simulink model "dsa2k_iwave_rfi"  (R2021a)
settings: Solver=VariableStepAuto  StartTime=0.0  StopTime=10.0  RelTol=1e-3
undefined symbols (not defined in the file): datetime, i, posixtime
libraries: xbsIndex_r4 x3053, casper_library_misc x61, rtr_casper_dsp_lib x31, xps_library x1
(part 4 of 43)

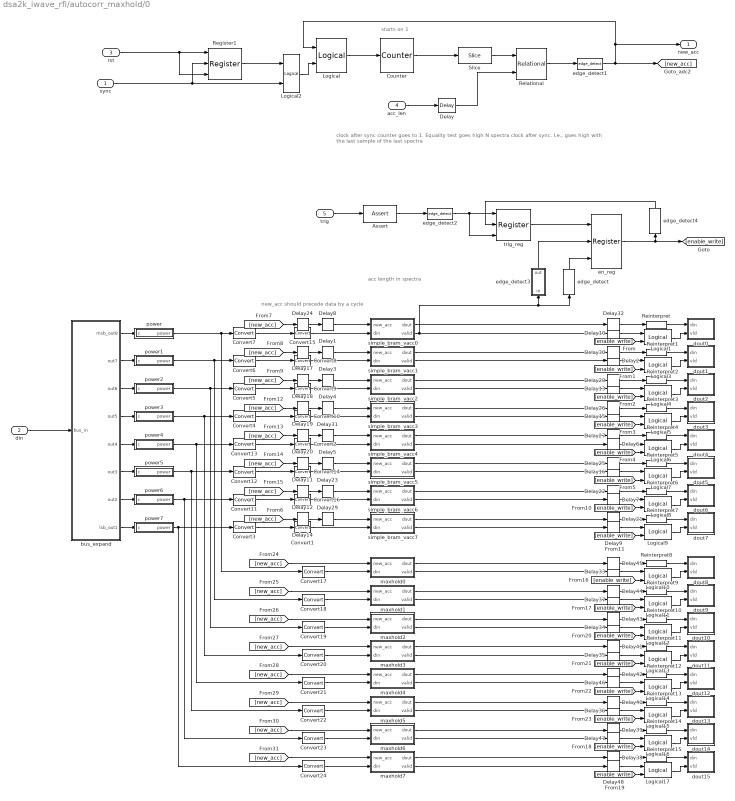
== system dsa2k_iwave_rfi/autocorr_maxhold/0 ==
  note: starts on 1
  note: clock after sync counter goes to 1.
      |
      | Equality test goes high N spectra clock after sync. I.e., goes high with the last sample of the last spectra
  note: acc length in spectra
  note: new_acc should precede data by a cycle
  sync : Inport
  din : Inport  Port=2
  rst : Inport  Port=3
  acc_len : Inport  Port=4
  trig : Inport  Port=5
  Assert : xbsIndex_r4/Assert  assert_type=off  type_source=Explicitly  gui_display_data_type=Fixed-point  arith_type="Signed  (2's comp)"  n_bits=16  bin_pt=14  preci_type=Single  exp_width=8  frac_width=24  assert_rate=on  rate_source=Explicitly  period=1  output_port=on  block_type=assert
  Convert{1..2,8..10,14..16} (8 alike) : xbsIndex_r4/Convert  gui_display_data_type=Floating-point  arith_type=Floating-point  n_bits=31  bin_pt=28  float_type=Single  exp_bits=8  fraction_bits=24  quantization="Round  (unbiased: Even Values)"  overflow=Wrap  en=off  latency=3  pipeline=on  dbl_ovrd=off  block_type=convert
  Convert{3..7,11..13} (8 alike) : xbsIndex_r4/Convert  gui_display_data_type=Fixed-point  arith_type="Signed  (2's comp)"  n_bits=37  bin_pt=34  float_type=Single  exp_bits=8  fraction_bits=24  quantization=Truncate  overflow=Wrap  en=off  latency=0  pipeline=off  dbl_ovrd=off  block_type=convert
  Convert{17..24} (8 alike) : xbsIndex_r4/Convert  gui_display_data_type=Fixed-point  arith_type=Unsigned  n_bits=32  bin_pt=30  float_type=Single  exp_bits=8  fraction_bits=24  quantization=Truncate  overflow=Wrap  en=off  latency=0  pipeline=off  dbl_ovrd=off  block_type=convert
  Counter : xbsIndex_r4/Counter  cnt_type=Free Running  cnt_to=Inf  operation=Up  start_count=1  cnt_by_val=1  arith_type=Unsigned  n_bits=30  bin_pt=0  load_pin=off  rst=on  en=off  explicit_period=on  period=1  use_behavioral_HDL=off  implementation=Fabric  dbl_ovrd=off  block_type=counter
  Delay{,2,6..7,9..10,13,15..16,33..37,46..48} (17 alike) : xbsIndex_r4/Delay  rst=off  infoeditControl=Selection of Reset will increase slice count due to use of real FFs and instead of SRLs  en=off  latency=1  reg_retiming=off  dbl_ovrd=off  block_type=delay
  Delay{1,3..5,8,23,29,31} (8 alike) : xbsIndex_r4/Delay  rst=off  infoeditControl=Selection of Reset will increase slice count due to use of real FFs and instead of SRLs  en=off  latency=4  reg_retiming=on  dbl_ovrd=off  block_type=delay
  Delay{11..12,14,17..20,24} (8 alike) : xbsIndex_r4/Delay  rst=off  infoeditControl=Selection of Reset will increase slice count due to use of real FFs and instead of SRLs  en=off  latency=3  reg_retiming=on  dbl_ovrd=off  block_type=delay
  Delay{21..22,25..28,30,32,38..45} (16 alike) : xbsIndex_r4/Delay  rst=off  infoeditControl=Selection of Reset will increase slice count due to use of real FFs and instead of SRLs  en=off  latency=1  reg_retiming=on  dbl_ovrd=off  block_type=delay
  Logical : xbsIndex_r4/Logical  logical_function=OR  inputs=2  en=off  latency=0  precision=Full  arith_type=Unsigned  n_bits=16  bin_pt=0  align_bp=on  dbl_ovrd=off  block_type=logical
  Logical{1..17} (17 alike) : xbsIndex_r4/Logical  logical_function=AND  inputs=2  en=off  latency=0  precision=Full  arith_type=Unsigned  n_bits=16  bin_pt=0  align_bp=on  dbl_ovrd=off  block_type=logical
  Register1 : xbsIndex_r4/Register  init=0  rst=on  en=on  dbl_ovrd=off  block_type=register
  Reinterpret{,1..15} (16 alike) : xbsIndex_r4/Reinterpret  force_arith_type=on  arith_type=Unsigned  force_bin_pt=on  bin_pt=0  block_type=reinterpret
  Relational : xbsIndex_r4/Relational  mode=a=b  op_type=Bool  en=off  latency=0  dbl_ovrd=off  block_type=relational
  Slice : xbsIndex_r4/Slice  nbits=30-nchan_bits-npol_bits  boolean_output=off  mode=Lower Bit Location + Width  bit1=0  base1=MSB of Input  bit0=nchan_bits + npol_bits  base0=LSB of Input  dbl_ovrd=off  block_type=slice
  bus_expand : Subsystem  AncestorBlock=casper_library_flow_control/bus_expand  mask(bus_expand){mode=divisions of equal size, outputNum=8, outputWidth=36, outputBinaryPt=0, outputArithmeticType=0, show_format=off, outputToWorkspace=off, variablePrefix=out, outputToModelAsWell=on}
      mask prompts: outputNum "Number of outputs:"; outputWidth "Output width:"; outputBinaryPt "Output binary point position:"; outputArithmeticType "Output arithmetic type (ufix=0, fix=1, bool=2):"; show_format "Print format string?"; outputToWorkspace "Output to workspace?"; variablePrefix "Variable name prefix:"; outputToModelAsWell "Output to model as well?"
      mask help:
      | Expands a 'bus' made using a bus_create or Xilinx
      | concat block.
      | The input will be divided into the specified number
      | of outputs with the specified arithmetic types.
      | Divisions are made from most significant bit.
      mask init: same as dsa2k_iwave_rfi/autocorr_maxhold/bus_expand
      settings: AttributesFormatString=8 outputs
      mask TypeOptions mode: divisions of equal size | divisions of arbitrary size
      mask Callback mode: %bus_expand_callback();
      mask Callback outputWidth: %bus_expand_callback();
      mask Callback outputToWorkspace: %bus_expand_callback();
  dout0 : Subsystem
  dout1 : Subsystem
  dout10 : Subsystem
  dout11 : Subsystem
  dout12 : Subsystem
  dout13 : Subsystem
  dout14 : Subsystem
  dout15 : Subsystem
  dout2 : Subsystem
  dout3 : Subsystem
  dout4 : Subsystem
  dout5 : Subsystem
  dout6 : Subsystem
  dout7 : Subsystem
  dout8 : Subsystem
  dout9 : Subsystem
  edge_detect{,1..2,4} (4 alike) : casper_library_misc/edge_detect  edge=Rising  polarity=Active High  x_in=[0 0.08 0.08 0.16 0.16 0.24 0.24 0.32 0.32 0.4]  y_in="[-1 -1  1  1  1  1  1  1  1  1]"  x_out=[0.6 0.68 0.68 0.76 0.76 0.84 0.84 0.92 0.92 1]  y_out="[-1 -1  1  1 -1 -1 -1 -1 -1 -1]"
  edge_detect3 : Subsystem  AncestorBlock=casper_library_misc/edge_detect  mask(edge_detect){edge=Falling, polarity=Active High, x_in=[0 0.08 0.08 0.16 0.16 0.24 0.24 0.32 0.32 0.4], y_in=[-1 -1  1  1  1  1  1  1  1  1], x_out=[0.6 0.68 0.68 0.76 0.76 0.84 0.84 0.92 0.92 1], y_out=[-1 -1  1  1 -1 -1 -1 -1 -1 -1]}
      mask prompts: edge "Edge Type"; polarity "Output Polarity"; x_in "Input X Positions"; y_in "Input Y Positions"; x_out "Output X Positions"; y_out "Output Y Positions"
      mask help: Output is active for one-cycle after each edge of the specified type (i.e. rising, falling or both).
      mask init: same as dsa2k_iwave_rfi/sync/ed1
      settings: AttributesFormatString=|
      | falling edges
      | active high
      mask Help: Output is active for one-cycle after each edge of the specified type (i.e. rising, falling, or both).  Latency is zero.
      mask TypeOptions edge: Rising | Falling | Both
      mask TypeOptions polarity: Active High | Active Low
      mask Display:
      | plot(x_in_num,0.5+y_in_num*0.2);
      | plot(x_out_num,0.5+y_out_num*0.2);
  en_reg : xbsIndex_r4/Register  init=0  rst=on  en=on  dbl_ovrd=off  block_type=register
  maxhold0 : Subsystem  AncestorBlock=casper_library_accumulators/simple_bram_vacc  mask(simple_bram_vacc){vec_len=2^(nchan_bits + npol_bits), arith_type=Unsigned, n_bits=32, bin_pt=30}
      mask prompts: vec_len "Vector length:"; arith_type "Output type:"; n_bits "Bit width (output):"; bin_pt "Binary point (output):"
      mask help: This simple vector accumulator is based on a shift register. It outputs its previous accumulated vector after a new_acc pulse is received.
      mask init:
      | % simple_bram_vacc_init(gcb, ...
      | %     'vec_len', vec_len, ...
      | %     'arith_type', arith_type, ...
      | %     'n_bits', n_bits, ...
      | %     'bin_pt', bin_pt);
      mask TypeOptions arith_type: Signed | Unsigned
  maxhold1 : Subsystem  AncestorBlock=casper_library_accumulators/simple_bram_vacc  mask(simple_bram_vacc){vec_len=2^(nchan_bits + npol_bits), arith_type=Unsigned, n_bits=32, bin_pt=30}
      mask prompts: vec_len "Vector length:"; arith_type "Output type:"; n_bits "Bit width (output):"; bin_pt "Binary point (output):"
      mask help: This simple vector accumulator is based on a shift register. It outputs its previous accumulated vector after a new_acc pulse is received.
      mask init:
      | % simple_bram_vacc_init(gcb, ...
      | %     'vec_len', vec_len, ...
      | %     'arith_type', arith_type, ...
      | %     'n_bits', n_bits, ...
      | %     'bin_pt', bin_pt);
      mask TypeOptions arith_type: Signed | Unsigned
  maxhold2 : Subsystem  AncestorBlock=casper_library_accumulators/simple_bram_vacc  mask(simple_bram_vacc){vec_len=2^(nchan_bits + npol_bits), arith_type=Unsigned, n_bits=32, bin_pt=30}
      mask prompts: vec_len "Vector length:"; arith_type "Output type:"; n_bits "Bit width (output):"; bin_pt "Binary point (output):"
      mask help: This simple vector accumulator is based on a shift register. It outputs its previous accumulated vector after a new_acc pulse is received.
      mask init:
      | % simple_bram_vacc_init(gcb, ...
      | %     'vec_len', vec_len, ...
      | %     'arith_type', arith_type, ...
      | %     'n_bits', n_bits, ...
      | %     'bin_pt', bin_pt);
      mask TypeOptions arith_type: Signed | Unsigned
  maxhold3 : Subsystem  AncestorBlock=casper_library_accumulators/simple_bram_vacc  mask(simple_bram_vacc){vec_len=2^(nchan_bits + npol_bits), arith_type=Unsigned, n_bits=32, bin_pt=30}
      mask prompts: vec_len "Vector length:"; arith_type "Output type:"; n_bits "Bit width (output):"; bin_pt "Binary point (output):"
      mask help: This simple vector accumulator is based on a shift register. It outputs its previous accumulated vector after a new_acc pulse is received.
      mask init:
      | % simple_bram_vacc_init(gcb, ...
      | %     'vec_len', vec_len, ...
      | %     'arith_type', arith_type, ...
      | %     'n_bits', n_bits, ...
      | %     'bin_pt', bin_pt);
      mask TypeOptions arith_type: Signed | Unsigned
  maxhold4 : Subsystem  AncestorBlock=casper_library_accumulators/simple_bram_vacc  mask(simple_bram_vacc){vec_len=2^(nchan_bits + npol_bits), arith_type=Unsigned, n_bits=32, bin_pt=30}
      mask prompts: vec_len "Vector length:"; arith_type "Output type:"; n_bits "Bit width (output):"; bin_pt "Binary point (output):"
      mask help: This simple vector accumulator is based on a shift register. It outputs its previous accumulated vector after a new_acc pulse is received.
      mask init:
      | % simple_bram_vacc_init(gcb, ...
      | %     'vec_len', vec_len, ...
      | %     'arith_type', arith_type, ...
      | %     'n_bits', n_bits, ...
      | %     'bin_pt', bin_pt);
      mask TypeOptions arith_type: Signed | Unsigned
  maxhold5 : Subsystem  AncestorBlock=casper_library_accumulators/simple_bram_vacc  mask(simple_bram_vacc){vec_len=2^(nchan_bits + npol_bits), arith_type=Unsigned, n_bits=32, bin_pt=30}
      mask prompts: vec_len "Vector length:"; arith_type "Output type:"; n_bits "Bit width (output):"; bin_pt "Binary point (output):"
      mask help: This simple vector accumulator is based on a shift register. It outputs its previous accumulated vector after a new_acc pulse is received.
      mask init:
      | % simple_bram_vacc_init(gcb, ...
      | %     'vec_len', vec_len, ...
      | %     'arith_type', arith_type, ...
      | %     'n_bits', n_bits, ...
      | %     'bin_pt', bin_pt);
      mask TypeOptions arith_type: Signed | Unsigned
  maxhold6 : Subsystem  AncestorBlock=casper_library_accumulators/simple_bram_vacc  mask(simple_bram_vacc){vec_len=2^(nchan_bits + npol_bits), arith_type=Unsigned, n_bits=32, bin_pt=30}
      mask prompts: vec_len "Vector length:"; arith_type "Output type:"; n_bits "Bit width (output):"; bin_pt "Binary point (output):"
      mask help: This simple vector accumulator is based on a shift register. It outputs its previous accumulated vector after a new_acc pulse is received.
      mask init:
      | % simple_bram_vacc_init(gcb, ...
      | %     'vec_len', vec_len, ...
      | %     'arith_type', arith_type, ...
      | %     'n_bits', n_bits, ...
      | %     'bin_pt', bin_pt);
      mask TypeOptions arith_type: Signed | Unsigned
  maxhold7 : Subsystem  AncestorBlock=casper_library_accumulators/simple_bram_vacc  mask(simple_bram_vacc){vec_len=2^(nchan_bits + npol_bits), arith_type=Unsigned, n_bits=32, bin_pt=30}
      mask prompts: vec_len "Vector length:"; arith_type "Output type:"; n_bits "Bit width (output):"; bin_pt "Binary point (output):"
      mask help: This simple vector accumulator is based on a shift register. It outputs its previous accumulated vector after a new_acc pulse is received.
      mask init:
      | % simple_bram_vacc_init(gcb, ...
      | %     'vec_len', vec_len, ...
      | %     'arith_type', arith_type, ...
      | %     'n_bits', n_bits, ...
      | %     'bin_pt', bin_pt);
      mask TypeOptions arith_type: Signed | Unsigned
  power : Subsystem  mask(power){BitWidth=18, add_latency=1, mult_latency=3}
      mask prompts: BitWidth "Bit Width"; add_latency "Add Latency"; mult_latency "Mult Latency"
      mask help: Squares real and imaginary components of complex input and adds them.
      mask Help: eval('xlWeb(''http://casper.berkeley.edu/wiki/Power'')')
      mask Display:
      | port_label('input', 1, 'c');
      | port_label('output', 1, 'power');
      | disp(['Z^-', num2str(mult_latency+add_latency)]);
  power1 : Subsystem  mask(power){BitWidth=18, add_latency=1, mult_latency=3}
      mask prompts: BitWidth "Bit Width"; add_latency "Add Latency"; mult_latency "Mult Latency"
      mask help: Squares real and imaginary components of complex input and adds them.
      mask Help: eval('xlWeb(''http://casper.berkeley.edu/wiki/Power'')')
      mask Display:
      | port_label('input', 1, 'c');
      | port_label('output', 1, 'power');
      | disp(['Z^-', num2str(mult_latency+add_latency)]);
  power2 : Subsystem  mask(power){BitWidth=18, add_latency=1, mult_latency=3}
      mask prompts: BitWidth "Bit Width"; add_latency "Add Latency"; mult_latency "Mult Latency"
      mask help: Squares real and imaginary components of complex input and adds them.
      mask Help: eval('xlWeb(''http://casper.berkeley.edu/wiki/Power'')')
      mask Display:
      | port_label('input', 1, 'c');
      | port_label('output', 1, 'power');
      | disp(['Z^-', num2str(mult_latency+add_latency)]);
  power3 : Subsystem  mask(power){BitWidth=18, add_latency=1, mult_latency=3}
      mask prompts: BitWidth "Bit Width"; add_latency "Add Latency"; mult_latency "Mult Latency"
      mask help: Squares real and imaginary components of complex input and adds them.
      mask Help: eval('xlWeb(''http://casper.berkeley.edu/wiki/Power'')')
      mask Display:
      | port_label('input', 1, 'c');
      | port_label('output', 1, 'power');
      | disp(['Z^-', num2str(mult_latency+add_latency)]);
  power4 : Subsystem  mask(power){BitWidth=18, add_latency=1, mult_latency=3}
      mask prompts: BitWidth "Bit Width"; add_latency "Add Latency"; mult_latency "Mult Latency"
      mask help: Squares real and imaginary components of complex input and adds them.
      mask Help: eval('xlWeb(''http://casper.berkeley.edu/wiki/Power'')')
      mask Display:
      | port_label('input', 1, 'c');
      | port_label('output', 1, 'power');
      | disp(['Z^-', num2str(mult_latency+add_latency)]);
  power5 : Subsystem  mask(power){BitWidth=18, add_latency=1, mult_latency=3}
      mask prompts: BitWidth "Bit Width"; add_latency "Add Latency"; mult_latency "Mult Latency"
      mask help: Squares real and imaginary components of complex input and adds them.
      mask Help: eval('xlWeb(''http://casper.berkeley.edu/wiki/Power'')')
      mask Display:
      | port_label('input', 1, 'c');
      | port_label('output', 1, 'power');
      | disp(['Z^-', num2str(mult_latency+add_latency)]);
  power6 : Subsystem  mask(power){BitWidth=18, add_latency=1, mult_latency=3}
      mask prompts: BitWidth "Bit Width"; add_latency "Add Latency"; mult_latency "Mult Latency"
      mask help: Squares real and imaginary components of complex input and adds them.
      mask Help: eval('xlWeb(''http://casper.berkeley.edu/wiki/Power'')')
      mask Display:
      | port_label('input', 1, 'c');
      | port_label('output', 1, 'power');
      | disp(['Z^-', num2str(mult_latency+add_latency)]);
  power7 : Subsystem  mask(power){BitWidth=18, add_latency=1, mult_latency=3}
      mask prompts: BitWidth "Bit Width"; add_latency "Add Latency"; mult_latency "Mult Latency"
      mask help: Squares real and imaginary components of complex input and adds them.
      mask Help: eval('xlWeb(''http://casper.berkeley.edu/wiki/Power'')')
      mask Display:
      | port_label('input', 1, 'c');
      | port_label('output', 1, 'power');
      | disp(['Z^-', num2str(mult_latency+add_latency)]);
  simple_bram_vacc0 : Subsystem  AncestorBlock=casper_library_accumulators/simple_bram_vacc  mask(simple_bram_vacc){vec_len=2^(nchan_bits + npol_bits), arith_type=Signed, n_bits=30 + 17, bin_pt=28}
      mask prompts: vec_len "Vector length:"; arith_type "Output type:"; n_bits "Bit width (output):"; bin_pt "Binary point (output):"
      mask help: This simple vector accumulator is based on a shift register. It outputs its previous accumulated vector after a new_acc pulse is received.
      mask init:
      | simple_bram_vacc_init(gcb, ...
      |     'vec_len', vec_len, ...
      |     'arith_type', arith_type, ...
      |     'n_bits', n_bits, ...
      |     'bin_pt', bin_pt);
      mask TypeOptions arith_type: Signed | Unsigned
  simple_bram_vacc1 : Subsystem  AncestorBlock=casper_library_accumulators/simple_bram_vacc  mask(simple_bram_vacc){vec_len=2^(nchan_bits + npol_bits), arith_type=Signed, n_bits=30 + 17, bin_pt=28}
      mask prompts: vec_len "Vector length:"; arith_type "Output type:"; n_bits "Bit width (output):"; bin_pt "Binary point (output):"
      mask help: This simple vector accumulator is based on a shift register. It outputs its previous accumulated vector after a new_acc pulse is received.
      mask init:
      | simple_bram_vacc_init(gcb, ...
      |     'vec_len', vec_len, ...
      |     'arith_type', arith_type, ...
      |     'n_bits', n_bits, ...
      |     'bin_pt', bin_pt);
      mask TypeOptions arith_type: Signed | Unsigned
  simple_bram_vacc2 : Subsystem  AncestorBlock=casper_library_accumulators/simple_bram_vacc  mask(simple_bram_vacc){vec_len=2^(nchan_bits + npol_bits), arith_type=Signed, n_bits=30 + 17, bin_pt=28}
      mask prompts: vec_len "Vector length:"; arith_type "Output type:"; n_bits "Bit width (output):"; bin_pt "Binary point (output):"
      mask help: This simple vector accumulator is based on a shift register. It outputs its previous accumulated vector after a new_acc pulse is received.
      mask init:
      | simple_bram_vacc_init(gcb, ...
      |     'vec_len', vec_len, ...
      |     'arith_type', arith_type, ...
      |     'n_bits', n_bits, ...
      |     'bin_pt', bin_pt);
      mask TypeOptions arith_type: Signed | Unsigned
  simple_bram_vacc3 : Subsystem  AncestorBlock=casper_library_accumulators/simple_bram_vacc  mask(simple_bram_vacc){vec_len=2^(nchan_bits + npol_bits), arith_type=Signed, n_bits=30 + 17, bin_pt=28}
      mask prompts: vec_len "Vector length:"; arith_type "Output type:"; n_bits "Bit width (output):"; bin_pt "Binary point (output):"
      mask help: This simple vector accumulator is based on a shift register. It outputs its previous accumulated vector after a new_acc pulse is received.
      mask init:
      | simple_bram_vacc_init(gcb, ...
      |     'vec_len', vec_len, ...
      |     'arith_type', arith_type, ...
      |     'n_bits', n_bits, ...
      |     'bin_pt', bin_pt);
      mask TypeOptions arith_type: Signed | Unsigned
  simple_bram_vacc4 : Subsystem  AncestorBlock=casper_library_accumulators/simple_bram_vacc  mask(simple_bram_vacc){vec_len=2^(nchan_bits + npol_bits), arith_type=Signed, n_bits=30 + 17, bin_pt=28}
      mask prompts: vec_len "Vector length:"; arith_type "Output type:"; n_bits "Bit width (output):"; bin_pt "Binary point (output):"
      mask help: This simple vector accumulator is based on a shift register. It outputs its previous accumulated vector after a new_acc pulse is received.
      mask init:
      | simple_bram_vacc_init(gcb, ...
      |     'vec_len', vec_len, ...
      |     'arith_type', arith_type, ...
      |     'n_bits', n_bits, ...
      |     'bin_pt', bin_pt);
      mask TypeOptions arith_type: Signed | Unsigned
  simple_bram_vacc5 : Subsystem  AncestorBlock=casper_library_accumulators/simple_bram_vacc  mask(simple_bram_vacc){vec_len=2^(nchan_bits + npol_bits), arith_type=Signed, n_bits=30 + 17, bin_pt=28}
      mask prompts: vec_len "Vector length:"; arith_type "Output type:"; n_bits "Bit width (output):"; bin_pt "Binary point (output):"
      mask help: This simple vector accumulator is based on a shift register. It outputs its previous accumulated vector after a new_acc pulse is received.
      mask init:
      | simple_bram_vacc_init(gcb, ...
      |     'vec_len', vec_len, ...
      |     'arith_type', arith_type, ...
      |     'n_bits', n_bits, ...
      |     'bin_pt', bin_pt);
      mask TypeOptions arith_type: Signed | Unsigned
  simple_bram_vacc6 : Subsystem  AncestorBlock=casper_library_accumulators/simple_bram_vacc  mask(simple_bram_vacc){vec_len=2^(nchan_bits + npol_bits), arith_type=Signed, n_bits=30 + 17, bin_pt=28}
      mask prompts: vec_len "Vector length:"; arith_type "Output type:"; n_bits "Bit width (output):"; bin_pt "Binary point (output):"
      mask help: This simple vector accumulator is based on a shift register. It outputs its previous accumulated vector after a new_acc pulse is received.
      mask init:
      | simple_bram_vacc_init(gcb, ...
      |     'vec_len', vec_len, ...
      |     'arith_type', arith_type, ...
      |     'n_bits', n_bits, ...
      |     'bin_pt', bin_pt);
      mask TypeOptions arith_type: Signed | Unsigned
  simple_bram_vacc7 : Subsystem  AncestorBlock=casper_library_accumulators/simple_bram_vacc  mask(simple_bram_vacc){vec_len=2^(nchan_bits + npol_bits), arith_type=Signed, n_bits=30 + 17, bin_pt=28}
      mask prompts: vec_len "Vector length:"; arith_type "Output type:"; n_bits "Bit width (output):"; bin_pt "Binary point (output):"
      mask help: This simple vector accumulator is based on a shift register. It outputs its previous accumulated vector after a new_acc pulse is received.
      mask init:
      | simple_bram_vacc_init(gcb, ...
      |     'vec_len', vec_len, ...
      |     'arith_type', arith_type, ...
      |     'n_bits', n_bits, ...
      |     'bin_pt', bin_pt);
      mask TypeOptions arith_type: Signed | Unsigned
  trig_reg : xbsIndex_r4/Register  init=0  rst=on  en=on  dbl_ovrd=off  block_type=register
  new_acc : Outport  VectorParamsAs1DForOutWhenUnconnected=off
  wires:
  Convert24/1 -> maxhold7/2(din)
  [new_acc] -> maxhold7/1(new_acc)
  [new_acc] -> maxhold6/1(new_acc)
  Convert23/1 -> maxhold6/2(din)
  Convert22/1 -> maxhold5/2(din)
  [new_acc] -> maxhold5/1(new_acc)
  [new_acc] -> maxhold4/1(new_acc)
  Convert21/1 -> maxhold4/2(din)
  Convert20/1 -> maxhold3/2(din)
  [new_acc] -> maxhold3/1(new_acc)
  Convert19/1 -> maxhold2/2(din)
  [new_acc] -> maxhold2/1(new_acc)
  Convert18/1 -> maxhold1/2(din)
  [new_acc] -> maxhold1/1(new_acc)
  Convert17/1 -> maxhold0/2(din)
  [new_acc] -> maxhold0/1(new_acc)
  Logical14/1 -> dout12/2(vld)
  [enable_write] -> Logical14/2
  [enable_write] -> Logical15/2
  Logical15/1 -> dout13/2(vld)
  Logical16/1 -> dout14/2(vld)
  [enable_write] -> Logical16/2
  [enable_write] -> Logical17/2
  Logical17/1 -> dout15/2(vld)
  maxhold4/1(dout) -> Delay42/1
  maxhold5/1(dout) -> Delay40/1
  maxhold6/1(dout) -> Delay39/1
  maxhold6/2(valid) -> Delay47/1
  maxhold7/1(dout) -> Delay38/1
  maxhold7/2(valid) -> Delay48/1
  maxhold5/2(valid) -> Delay36/1
  maxhold4/2(valid) -> Delay46/1
  Delay42/1 -> Reinterpret12/1
  Delay46/1 -> Logical14/1
  Delay40/1 -> Reinterpret13/1
  Delay36/1 -> Logical15/1
  Delay39/1 -> Reinterpret14/1
  Delay47/1 -> Logical16/1
  Delay48/1 -> Logical17/1
  Delay38/1 -> Reinterpret15/1
  Reinterpret12/1 -> dout12/1(din)
  Reinterpret13/1 -> dout13/1(din)
  Reinterpret14/1 -> dout14/1(din)
  Reinterpret15/1 -> dout15/1(din)
  Reinterpret11/1 -> dout11/1(din)
  Reinterpret10/1 -> dout10/1(din)
  Reinterpret9/1 -> dout9/1(din)
  Reinterpret8/1 -> dout8/1(din)
  Delay41/1 -> Reinterpret11/1
  Delay35/1 -> Logical13/1
  Delay34/1 -> Logical12/1
  Delay43/1 -> Reinterpret10/1
  Delay37/1 -> Logical11/1
  Delay44/1 -> Reinterpret9/1
  Delay33/1 -> Logical10/1
  Delay45/1 -> Reinterpret8/1
  maxhold0/2(valid) -> Delay33/1
  maxhold1/2(valid) -> Delay37/1
  maxhold3/2(valid) -> Delay35/1
  maxhold3/1(dout) -> Delay41/1
  maxhold2/2(valid) -> Delay34/1
  maxhold2/1(dout) -> Delay43/1
  maxhold1/1(dout) -> Delay44/1
  maxhold0/1(dout) -> Delay45/1
  Logical13/1 -> dout11/2(vld)
  [enable_write] -> Logical13/2
  [enable_write] -> Logical12/2
  Logical12/1 -> dout10/2(vld)
  Logical11/1 -> dout9/2(vld)
  [enable_write] -> Logical11/2
  [enable_write] -> Logical10/2
  Logical10/1 -> dout8/2(vld)
  bus_expand/8(lsb_out1) -> power7/1(c)
  bus_expand/7(out2) -> power6/1(c)
  bus_expand/6(out3) -> power5/1(c)
  bus_expand/5(out4) -> power4/1(c)
  bus_expand/4(out5) -> power3/1(c)
  bus_expand/3(out6) -> power2/1(c)
  bus_expand/2(out7) -> power1/1(c)
  bus_expand/1(msb_out8) -> power/1(c)
  Delay/1 -> Relational/2
  Delay8/1 -> simple_bram_vacc0/1(new_acc)
  Delay1/1 -> simple_bram_vacc1/1(new_acc)
  Delay3/1 -> simple_bram_vacc2/1(new_acc)
  Delay4/1 -> simple_bram_vacc3/1(new_acc)
  acc_len/1 -> Delay/1
  Logical2/1 -> Logical/2
  Relational/1 -> edge_detect1/1
  Slice/1 -> Relational/1
  din/1 -> bus_expand/1(bus_in)
  power3/1(power) -> Convert20/1, Convert4/1
  power2/1(power) -> Convert19/1, Convert5/1
  power1/1(power) -> Convert18/1, Convert6/1
  power/1(power) -> Convert7/1, Convert17/1
  [new_acc] -> Delay19/1
  [new_acc] -> Delay18/1
  [new_acc] -> Delay17/1
  [new_acc] -> Delay24/1
  Counter/1 -> Slice/1
  Logical/1 -> Counter/1
  edge_detect1/1 -> [new_acc], new_acc/1, Logical/1
  rst/1 -> Register1/1, Register1/3
  Register1/1 -> Logical2/1
  sync/1 -> Logical2/2, Register1/2
  trig_reg/1 -> en_reg/1
  edge_detect2/1 -> trig_reg/3, trig_reg/1
  edge_detect/1 -> en_reg/3
  edge_detect3/1(out) -> en_reg/2
  edge_detect4/1 -> trig_reg/2
  Logical1/1 -> dout0/2(vld)
  en_reg/1 -> [enable_write], edge_detect4/1
  [enable_write] -> Logical1/2
  [enable_write] -> Logical3/2
  Logical3/1 -> dout1/2(vld)
  Logical4/1 -> dout2/2(vld)
  [enable_write] -> Logical4/2
  [enable_write] -> Logical5/2
  Logical5/1 -> dout3/2(vld)
  trig/1 -> Assert/1
  Assert/1 -> edge_detect2/1
  simple_bram_vacc0/1(dout) -> Delay32/1
  simple_bram_vacc1/1(dout) -> Delay30/1
  simple_bram_vacc2/1(dout) -> Delay28/1
  simple_bram_vacc2/2(valid) -> Delay13/1
  simple_bram_vacc3/1(dout) -> Delay26/1
  simple_bram_vacc3/2(valid) -> Delay15/1
  simple_bram_vacc1/2(valid) -> Delay2/1
  simple_bram_vacc0/2(valid) -> Delay10/1, edge_detect/1, edge_detect3/1(in)
  Delay19/1 -> Delay4/1
  Convert10/1 -> simple_bram_vacc3/2(din)
  Delay18/1 -> Delay3/1
  Convert9/1 -> simple_bram_vacc2/2(din)
  Convert8/1 -> simple_bram_vacc1/2(din)
  Delay17/1 -> Delay1/1
  Delay24/1 -> Delay8/1
  Convert15/1 -> simple_bram_vacc0/2(din)
  Delay32/1 -> Reinterpret/1
  Delay10/1 -> Logical1/1
  Delay30/1 -> Reinterpret1/1
  Delay2/1 -> Logical3/1
  Delay28/1 -> Reinterpret2/1
  Delay13/1 -> Logical4/1
  Delay15/1 -> Logical5/1
  Delay26/1 -> Reinterpret3/1
  Convert4/1 -> Convert10/1
  Convert5/1 -> Convert9/1
  Convert6/1 -> Convert8/1
  Convert7/1 -> Convert15/1
  Reinterpret/1 -> dout0/1(din)
  Reinterpret1/1 -> dout1/1(din)
  Reinterpret2/1 -> dout2/1(din)
  Reinterpret3/1 -> dout3/1(din)
  Reinterpret7/1 -> dout7/1(din)
  Reinterpret6/1 -> dout6/1(din)
  Reinterpret5/1 -> dout5/1(din)
  Reinterpret4/1 -> dout4/1(din)
  Convert13/1 -> Convert2/1
  Convert12/1 -> Convert14/1
  Convert11/1 -> Convert16/1
  Convert3/1 -> Convert1/1
  Delay21/1 -> Reinterpret7/1
  Delay9/1 -> Logical9/1
  Delay7/1 -> Logical8/1
  Delay22/1 -> Reinterpret6/1
  Delay16/1 -> Logical7/1
  Delay25/1 -> Reinterpret5/1
  Delay6/1 -> Logical6/1
  Delay27/1 -> Reinterpret4/1
  Convert2/1 -> simple_bram_vacc4/2(din)
  Delay20/1 -> Delay31/1
  Delay11/1 -> Delay5/1
  Convert14/1 -> simple_bram_vacc5/2(din)
  Convert16/1 -> simple_bram_vacc6/2(din)
  Delay12/1 -> Delay23/1
  Convert1/1 -> simple_bram_vacc7/2(din)
  Delay14/1 -> Delay29/1
  simple_bram_vacc4/2(valid) -> Delay6/1
  simple_bram_vacc5/2(valid) -> Delay16/1
  simple_bram_vacc7/2(valid) -> Delay9/1
  simple_bram_vacc7/1(dout) -> Delay21/1
  simple_bram_vacc6/2(valid) -> Delay7/1
  simple_bram_vacc6/1(dout) -> Delay22/1
  simple_bram_vacc5/1(dout) -> Delay25/1
  simple_bram_vacc4/1(dout) -> Delay27/1
  Logical9/1 -> dout7/2(vld)
  [enable_write] -> Logical9/2
  [enable_write] -> Logical8/2
  Logical8/1 -> dout6/2(vld)
  Logical7/1 -> dout5/2(vld)
  [enable_write] -> Logical7/2
  [enable_write] -> Logical6/2
  Logical6/1 -> dout4/2(vld)
  [new_acc] -> Delay20/1
  [new_acc] -> Delay11/1
  [new_acc] -> Delay12/1
  [new_acc] -> Delay14/1
  power4/1(power) -> Convert21/1, Convert13/1
  power5/1(power) -> Convert22/1, Convert12/1
  power6/1(power) -> Convert23/1, Convert11/1
  power7/1(power) -> Convert24/1, Convert3/1
  Delay29/1 -> simple_bram_vacc7/1(new_acc)
  Delay23/1 -> simple_bram_vacc6/1(new_acc)
  Delay5/1 -> simple_bram_vacc5/1(new_acc)
  Delay31/1 -> simple_bram_vacc4/1(new_acc)
